simulink model "SystemModel"  (R2026a)
settings: Solver=FixedStepDiscrete  StopTime=inf  FixedStep=ts_system  EnableMultiTasking=on
StartFcn:
  | Simulink.sdi.setRecordData(false);
undefined symbols (not defined in the file): Battery, BCE12, BCE_Set_init, BMS_Controller_State, Cell10_P, Cell11_P, Cell12_P, Cell1_N, Cell1_P, Cell2_P, Cell3_P, Cell4_P, Cell5_P, Cell6_P, Cell7_P, Cell8_P, Cell9_P, Cell_Temperatures, Cell_Voltages, Charging_State, currentFactor, CV_Gain, Device_01, DiscIntNeverNeededParam, I_cc, MaxCellVoltThrsld, noCurrent, Ns_Module, NumModules, OverCellVoltageLimit, sg_bce, SOCInit, SRE, ts_controller, ts_system, UnderCellVoltageLimit, voltThreshold
libraries: slrealtimeethercatlib x99, fl_lib x65, nesl_utility x43, simulink x23, slrealtimeutilitieslib x13, sl_discontinuities x13, dspstat3 x12, canmsglib x11, speedgoatlib_IO611 x9, batt_lib x3, sharedTrackingLibrary x2, BatteryModuleLibrary_12Cells_lib x1
(part 5 of 6)

== system SystemModel/BMS/MIL/Controller/Current Calculations/Discharge_Current_Limit_Calc ==
  MinCellVolt : Inport
  MinCellTemp : Inport  Port=2
  MaxCellTemp : Inport  Port=3
  Divide : Product  Inputs=*/
  Gain : Gain  Gain=-1
  HighTempDchrgCurrentLim : Lookup_n-D  NumberOfTableDimensions=1  BreakpointsForDimension1=273.15+[-30:1:70]  Table=100*(1-tanh(273.15+[-30:1:70]-273.15-50))/2  InternalRulePriority=Speed  RndMeth=Simplest
  InternalCellResistance : Constant  Value=single(max(max(Battery(1).R0_LUT)))  OutDataTypeStr=single  SampleTime=-1
  LowTempDchrgCurrentLim : Lookup_n-D  NumberOfTableDimensions=1  BreakpointsForDimension1=273.15+[-30:1:70]  Table=100*(1+tanh(273.15+[-30:1:70]-(273.15)))/2  InternalRulePriority=Speed  RndMeth=Simplest
  MinMax2 : MinMax  Inputs=3
  Subtract : Sum  Inputs=+-
  UnderVoltageLimit : Constant  Value=UnderCellVoltageLimit  OutDataTypeStr=single  SampleTime=-1
  Discharge_Current_Limit : Outport  VectorParamsAs1DForOutWhenUnconnected=off
  wires:
  MinMax2/1 -> Gain/1  "DischargeCurrentLimit"
  Divide/1 -> MinMax2/1
  MinCellVolt/1 -> Subtract/1
  InternalCellResistance/1 -> Divide/2
  Subtract/1 -> Divide/1
  UnderVoltageLimit/1 -> Subtract/2
  Gain/1 -> Discharge_Current_Limit/1
  MaxCellTemp/1 -> HighTempDchrgCurrentLim/1
  MinCellTemp/1 -> LowTempDchrgCurrentLim/1
  HighTempDchrgCurrentLim/1 -> MinMax2/3
  LowTempDchrgCurrentLim/1 -> MinMax2/2

== system SystemModel/BMS/MIL/Controller/SOC Calculation/Coulomb Counting ==
  Curr : Inport
  Temp : Inport  Port=2
  1-D Lookup Table : Lookup_n-D  NumberOfTableDimensions=1  BreakpointsForDimension1=single(Battery(1).Temperature_LUT)  Table=single(Battery(1).Capacity_LUT)  InternalRulePriority=Speed  RndMeth=Simplest
  Discrete-Time Integrator : DiscreteIntegrator  InitialCondition=single(SOCInit+0.05)  SampleTime=-1  LimitOutput=on  UpperSaturationLimit=1  LowerSaturationLimit=0  ICPrevOutput=DiscIntNeverNeededParam  ICPrevScaledInput=DiscIntNeverNeededParam
  Divide : Product  Inputs=*/
  Gain : Gain  Gain=single(1/3600)
  SOC : Outport  VectorParamsAs1DForOutWhenUnconnected=off
  wires:
  Discrete-Time Integrator/1 -> SOC/1
  Curr/1 -> Gain/1
  Gain/1 -> Divide/1
  Divide/1 -> Discrete-Time Integrator/1
  1-D Lookup Table/1 -> Divide/2  "Capacity"
  Temp/1 -> 1-D Lookup Table/1

== system SystemModel/BMS/MIL/Controller/SOC Calculation/Measurement Function ==
  Current : Inport
  Temperature (K) : Inport  Port=2
  batteryMeasurementFcn : TriggerPort  TriggerType=function-call  IsSimulinkFunction=on  FunctionName=batteryMeasurementFcn  VariantControl=Variant
  Add1 : Sum  Inputs=+--
  Em Table : Lookup_n-D  BreakpointsForDimension1=Battery.SOC_LUT  BreakpointsForDimension2=Battery.Temperature_LUT  BeginIndexSearchUsingPreviousIndexResult=on  Table=Battery.Em_LUT  ExtrapMethod=Clip  InternalRulePriority=Speed  RndMeth=Simplest
      settings: InputPortMap=u0,u1
  Get SOC : Selector  InputPortWidth=2  IndexOptions=Index vector (dialog)  Indices=[1]  OutputSizes=1
  Get U1 : Selector  InputPortWidth=2  IndexOptions=Index vector (dialog)  Indices=2  OutputSizes=1
  Product : Product
  R0 Table : Lookup_n-D  BreakpointsForDimension1=Battery.SOC_LUT  BreakpointsForDimension2=Battery.Temperature_LUT  BeginIndexSearchUsingPreviousIndexResult=on  Table=Battery.R0_LUT  ExtrapMethod=Clip  InternalRulePriority=Speed  RndMeth=Simplest
      settings: InputPortMap=u0,u1
  x : ArgIn  DisableCoverage=on  OutDataTypeStr=single  PortDimensions=2  ArgumentName=x
  y : ArgOut  DisableCoverage=on  OutDataTypeStr=single  ArgumentName=y
  wires:
  Get U1/1 -> Add1/3  "U1"
  Product/1 -> Add1/2
  Current/1 -> Product/2
  R0 Table/1 -> Product/1
  Temperature (K)/1 -> Em Table/2, R0 Table/2
  Add1/1 -> y/1
  Em Table/1 -> Add1/1
  Get SOC/1 -> Em Table/1, R0 Table/1  "SOC"
  x/1 -> Get SOC/1, Get U1/1

== system SystemModel/BMS/MIL/Controller/SOC Calculation/State Transition Function ==
  Current : Inport
  Temperature K : Inport  Port=2
  batteryStateFcn : TriggerPort  TriggerType=function-call  IsSimulinkFunction=on  FunctionName=batteryStateFcn  VariantControl=Variant
  Add : Sum
  Add1 : Sum  Inputs=-+
  C1 : Lookup_n-D  BreakpointsForDimension1=Battery.SOC_LUT  BreakpointsForDimension2=Battery.Temperature_LUT  BeginIndexSearchUsingPreviousIndexResult=on  Table=Battery.C1_LUT  ExtrapMethod=Clip  InternalRulePriority=Speed  RndMeth=Simplest
      settings: InputPortMap=u0,u1
  Constant : Constant  Value=single(ts_system)  OutDataTypeStr=single
  Divide : Product  Inputs=*/
  Divide1 : Product  Inputs=*/
  Divide2 : Product  Inputs=*/
  Gain : Gain  Gain=-3600
  Get SOC : Selector  InputPortWidth=2  IndexOptions=Index vector (dialog)  Indices=1  OutputSizes=1
  Get U1 : Selector  InputPortWidth=2  IndexOptions=Index vector (dialog)  Indices=2  OutputSizes=1
  Lookup Table : Lookup_n-D  NumberOfTableDimensions=1  BreakpointsForDimension1=Battery.Temperature_LUT  BeginIndexSearchUsingPreviousIndexResult=on  Table=Battery.Capacity_LUT  InternalRulePriority=Speed  RndMeth=Simplest
  Mux : Mux  Inputs=2
  Product : Product  OutDataTypeStr=single
  Product1 : Product
  R1 : Lookup_n-D  BreakpointsForDimension1=Battery.SOC_LUT  BreakpointsForDimension2=Battery.Temperature_LUT  BeginIndexSearchUsingPreviousIndexResult=on  Table=Battery.R1_LUT  ExtrapMethod=Clip  InternalRulePriority=Speed  RndMeth=Simplest
      settings: InputPortMap=u0,u1
  x : ArgIn  DisableCoverage=on  OutDataTypeStr=single  PortDimensions=2  ArgumentName=x
  xNext : ArgOut  DisableCoverage=on  OutDataTypeStr=single  PortDimensions=2  ArgumentName=xNext
  wires:
  Lookup Table/1 -> Gain/1  "Cq"
  Product/1 -> Add/2
  Constant/1 -> Product/2
  Current/1 -> Divide1/1, Divide/1  "Current"
  Get SOC/1 -> C1/1, R1/1
  Temperature K/1 -> Lookup Table/1, C1/2, R1/2
  Add/1 -> xNext/1
  x/1 -> Add/1, Get U1/1, Get SOC/1
  Gain/1 -> Divide/2
  Divide/1 -> Mux/1  "xdot_1"
  Get U1/1 -> Divide2/1  "U1"
  Product1/1 -> Divide2/2  "R1*C1"
  R1/1 -> Product1/1  "R1"
  C1/1 -> Product1/2, Divide1/2  "C1"
  Divide1/1 -> Add1/2  "Current/C1"
  Divide2/1 -> Add1/1
  Add1/1 -> Mux/2  "xdot_2"
  Mux/1 -> Product/1  "xdot"

== system SystemModel/BMS/MIL/Controller/SOC Calculation/UKF_EKF_1TC ==
  Cell_Voltage : Inport
  Enable : EnablePort
  EKF : sharedTrackingLibrary/Extended Kalman Filter  StateTransitionFcn=batteryStateFcn  HasStateTransitionJacobianFcn=off  HasAdditiveProcessNoise=Additive  ProcessNoise=1e-10*eye(2)  HasTimeVaryingProcessNoise=off  HasStateTransitionFcnExtraArgument=0  InitialState=[single(SOCInit+0.05); 0;]  InitialStateCovariance=[1e-5 1]  MeasurementFcn1=batteryMeasurementFcn  HasMeasurementJacobianFcn1=off  HasMeasurementEnablePort1=off  HasAdditiveMeasurementNoise1=Additive  MeasurementNoise1=1e-1  HasTimeVaryingMeasurementNoise1=off  HasMeasurementFcnExtraArgument1=0  HasMeasurementWrapping1=off  MeasurementFcn2=myMeasurementFcn  HasMeasurementJacobianFcn2=off  HasMeasurementEnablePort2=off  HasAdditiveMeasurementNoise2=Additive  MeasurementNoise2=1  HasTimeVaryingMeasurementNoise2=off  HasMeasurementFcnExtraArgument2=0  HasMeasurementWrapping2=off  MeasurementFcn3=myMeasurementFcn  HasMeasurementJacobianFcn3=off  HasMeasurementEnablePort3=off  HasAdditiveMeasurementNoise3=Additive  MeasurementNoise3=1  HasTimeVaryingMeasurementNoise3=off  HasMeasurementFcnExtraArgument3=0  HasMeasurementWrapping3=off  MeasurementFcn4=myMeasurementFcn  HasMeasurementJacobianFcn4=off  HasMeasurementEnablePort4=off  HasAdditiveMeasurementNoise4=Additive  MeasurementNoise4=1  HasTimeVaryingMeasurementNoise4=off  HasMeasurementFcnExtraArgument4=0  HasMeasurementWrapping4=off  MeasurementFcn5=myMeasurementFcn  HasMeasurementJacobianFcn5=off  HasMeasurementEnablePort5=off  HasAdditiveMeasurementNoise5=Additive  MeasurementNoise5=1  HasTimeVaryingMeasurementNoise5=off  HasMeasurementFcnExtraArgument5=0  HasMeasurementWrapping5=off  EnableMultirate=off  StateTransitionFcnSampleTime=1  MeasurementFcn1SampleTime=1  MeasurementFcn2SampleTime=1  MeasurementFcn3SampleTime=1  MeasurementFcn4SampleTime=1  MeasurementFcn5SampleTime=1  UseCurrentEstimator=on  OutputStateCovariance=off  DataType=single  SampleTime=ts_controller  NumberOfMeasurements=1
  SOC : Selector  InputPortWidth=2  IndexOptions=Index vector (dialog)  Indices=1  OutputSizes=1
  SOC1 : Selector  InputPortWidth=2  IndexOptions=Index vector (dialog)  Indices=1  OutputSizes=1
  UKF : sharedTrackingLibrary/Unscented Kalman Filter  StateTransitionFcn=batteryStateFcn  HasAdditiveProcessNoise=Additive  ProcessNoise=1e-10*eye(2)  HasTimeVaryingProcessNoise=off  HasStateTransitionFcnExtraArgument=0  InitialState=[single(SOCInit+0.05); 0;]  InitialStateCovariance=[1e-5 1]  Alpha=1  Beta=2  Kappa=1  MeasurementFcn1=batteryMeasurementFcn  HasMeasurementEnablePort1=off  HasAdditiveMeasurementNoise1=Additive  MeasurementNoise1=0.1  HasTimeVaryingMeasurementNoise1=off  HasMeasurementFcnExtraArgument1=0  HasMeasurementWrapping1=off  MeasurementFcn2=myMeasurementFcn  HasMeasurementEnablePort2=off  HasAdditiveMeasurementNoise2=Additive  MeasurementNoise2=1  HasTimeVaryingMeasurementNoise2=off  HasMeasurementFcnExtraArgument2=0  HasMeasurementWrapping2=off  MeasurementFcn3=myMeasurementFcn  HasMeasurementEnablePort3=off  HasAdditiveMeasurementNoise3=Additive  MeasurementNoise3=1  HasTimeVaryingMeasurementNoise3=off  HasMeasurementFcnExtraArgument3=0  HasMeasurementWrapping3=off  MeasurementFcn4=myMeasurementFcn  HasMeasurementEnablePort4=off  HasAdditiveMeasurementNoise4=Additive  MeasurementNoise4=1  HasTimeVaryingMeasurementNoise4=off  HasMeasurementFcnExtraArgument4=0  HasMeasurementWrapping4=off  MeasurementFcn5=myMeasurementFcn  HasMeasurementEnablePort5=off  HasAdditiveMeasurementNoise5=Additive  MeasurementNoise5=1  HasTimeVaryingMeasurementNoise5=off  HasMeasurementFcnExtraArgument5=0  HasMeasurementWrapping5=off  EnableMultirate=off  StateTransitionFcnSampleTime=-1  MeasurementFcn1SampleTime=-1  MeasurementFcn2SampleTime=-1  MeasurementFcn3SampleTime=-1  MeasurementFcn4SampleTime=-1  MeasurementFcn5SampleTime=-1  UseCurrentEstimator=on  OutputStateCovariance=off  DataType=single  SampleTime=ts_controller  NumberOfMeasurements=1
  SOC_UKF : Outport  VectorParamsAs1DForOutWhenUnconnected=off
  SOC_EKF : Outport  Port=2  VectorParamsAs1DForOutWhenUnconnected=off
  wires:
  UKF/1 -> SOC1/1
  Cell_Voltage/1 -> UKF/1, EKF/1
  SOC1/1 -> SOC_UKF/1  "SOC_UKF"
  EKF/1 -> SOC/1
  SOC/1 -> SOC_EKF/1  "SOC_EKF"

== system SystemModel/Battery/Bypass/Bypass Values/12-Cell/Celsius_to_Kelvin ==
  C : Inport
  Add : Sum
  Constant : Constant  Value=273.15  SampleTime=-1
  Data Type Conversion3 : DataTypeConversion  OutDataTypeStr=single  SaturateOnIntegerOverflow=off  RndMeth=Floor
  K : Outport
  wires:
  Constant/1 -> Add/2
  Add/1 -> Data Type Conversion3/1
  C/1 -> Add/1
  Data Type Conversion3/1 -> K/1  "LowTempLimit"

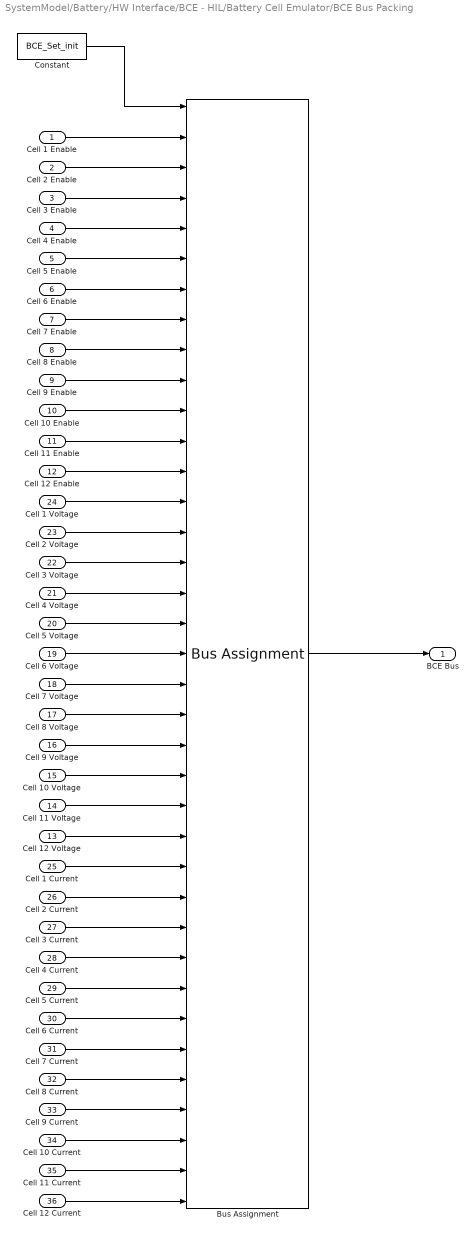
== system SystemModel/Battery/HW Interface/BCE - HIL/Battery Cell Emulator/BCE Bus Packing  ==
  Cell 1 Enable : Inport
  Cell 2 Enable : Inport  Port=2
  Cell 3 Enable : Inport  Port=3
  Cell 4 Enable : Inport  Port=4
  Cell 5 Enable : Inport  Port=5
  Cell 6 Enable : Inport  Port=6
  Cell 7 Enable : Inport  Port=7
  Cell 8 Enable : Inport  Port=8
  Cell 9 Enable : Inport  Port=9
  Cell 10 Enable : Inport  Port=10
  Cell 11 Enable : Inport  Port=11
  Cell 12 Enable : Inport  Port=12
  Cell 12 Voltage : Inport  Port=13
  Cell 11 Voltage : Inport  Port=14
  Cell 10 Voltage : Inport  Port=15
  Cell 9 Voltage : Inport  Port=16
  Cell 8 Voltage : Inport  Port=17
  Cell 7 Voltage : Inport  Port=18
  Cell 6 Voltage : Inport  Port=19
  Cell 5 Voltage : Inport  Port=20
  Cell 4 Voltage : Inport  Port=21
  Cell 3 Voltage : Inport  Port=22
  Cell 2 Voltage : Inport  Port=23
  Cell 1 Voltage : Inport  Port=24
  Cell 1 Current : Inport  Port=25
  Cell 2 Current : Inport  Port=26
  Cell 3 Current : Inport  Port=27
  Cell 4 Current : Inport  Port=28
  Cell 5 Current : Inport  Port=29
  Cell 6 Current : Inport  Port=30
  Cell 7 Current : Inport  Port=31
  Cell 8 Current : Inport  Port=32
  Cell 9 Current : Inport  Port=33
  Cell 10 Current : Inport  Port=34
  Cell 11 Current : Inport  Port=35
  Cell 12 Current : Inport  Port=36
  Bus Assignment : BusAssignment  AssignedSignals=Cell_1.Enable,Cell_2.Enable,Cell_3.Enable,Cell_4.Enable,Cell_5.Enable,Cell_6.Enable,Cell_7.Enable,Cell_8.Enable,Cell_9.Enable,Cell_10.Enable,Cell_11.Enable,Cell_12.Enable,Cell_1.V,Cell_2.V,Cell_3.V,Cell_4.V,Cell_5.V,Cell_6.V,Cell_7.V,Cell_8.V,Cell_9.V,Cell_10.V,Cell_11.V,Cell_12.V,Cell_1.I,Cell_2.I,Cell_3.I,Cell_4.I,Cell_5.I,Cell_6.I,Cell_7.I,Cell_8.I,Cell_9.I,Cell_10.I,Cell_11.I,Cell_12.I
  Constant : Constant  Value=BCE_Set_init  OutDataTypeStr=Bus: BCE_Set
  BCE Bus : Outport
  wires:
  Cell 11 Enable/1 -> Bus Assignment/12
  Cell 11 Voltage/1 -> Bus Assignment/24
  Cell 11 Current/1 -> Bus Assignment/36
  Cell 12 Current/1 -> Bus Assignment/37
  Cell 12 Voltage/1 -> Bus Assignment/25
  Cell 12 Enable/1 -> Bus Assignment/13
  Cell 10 Enable/1 -> Bus Assignment/11
  Cell 10 Voltage/1 -> Bus Assignment/23
  Cell 10 Current/1 -> Bus Assignment/35
  Cell 9 Current/1 -> Bus Assignment/34
  Cell 9 Voltage/1 -> Bus Assignment/22
  Cell 9 Enable/1 -> Bus Assignment/10
  Cell 5 Enable/1 -> Bus Assignment/6
  Cell 5 Voltage/1 -> Bus Assignment/18
  Cell 5 Current/1 -> Bus Assignment/30
  Cell 6 Current/1 -> Bus Assignment/31
  Cell 6 Voltage/1 -> Bus Assignment/19
  Cell 6 Enable/1 -> Bus Assignment/7
  Cell 8 Enable/1 -> Bus Assignment/9
  Cell 8 Voltage/1 -> Bus Assignment/21
  Cell 8 Current/1 -> Bus Assignment/33
  Cell 7 Current/1 -> Bus Assignment/32
  Cell 7 Voltage/1 -> Bus Assignment/20
  Cell 7 Enable/1 -> Bus Assignment/8
  Cell 3 Enable/1 -> Bus Assignment/4
  Cell 3 Voltage/1 -> Bus Assignment/16
  Cell 3 Current/1 -> Bus Assignment/28
  Cell 4 Current/1 -> Bus Assignment/29
  Cell 4 Voltage/1 -> Bus Assignment/17
  Cell 4 Enable/1 -> Bus Assignment/5
  Cell 2 Enable/1 -> Bus Assignment/3
  Cell 2 Voltage/1 -> Bus Assignment/15
  Cell 2 Current/1 -> Bus Assignment/27
  Cell 1 Current/1 -> Bus Assignment/26
  Cell 1 Enable/1 -> Bus Assignment/2
  Bus Assignment/1 -> BCE Bus/1
  Constant/1 -> Bus Assignment/1
  Cell 1 Voltage/1 -> Bus Assignment/14

== system SystemModel/Battery/HW Interface/BCE - HIL/Battery Cell Emulator/BCE Read  ==
  Subsystem : Subsystem
  Data : Outport  OutDataTypeStr=Bus: BCE_Get
  wires:
  Subsystem/1(Data) -> Data/1

== system SystemModel/Battery/HW Interface/BCE - HIL/Battery Cell Emulator/BCE Setup  ==
  EtherCAT Init : slrealtimeethercatlib/EtherCAT Init  Priority=0  config_file=C:\Users\jatin.anand\AppData\Local\Temp\sg_bmts\SystemModel\sg_bmts_ENI_bus0.xml  device_id=0  portnum=1  initstate=2  dctuning=0  enaDebug=0  logFile='c:\dbglog.txt'  sample_time=0.001000  DCMode=0
  Terminator : Terminator
  wires:
  EtherCAT Init/1 -> Terminator/1

== system SystemModel/Battery/HW Interface/BCE - HIL/Battery Cell Emulator/BCE Write  ==
  Data : Inport  OutDataTypeStr=Bus: BCE_Set
  Subsystem : Subsystem
  wires:
  Data/1 -> Subsystem/1(Data)

== system SystemModel/Battery/HW Interface/BCE - HIL/Battery Cell Emulator/BCE Read /Subsystem ==
  "BCE Read " : Subsystem
  Data : Outport  OutDataTypeStr=Bus: BCE_Get
  wires:
  "BCE Read "/1(Data) -> Data/1

== system SystemModel/Battery/HW Interface/BCE - HIL/Battery Cell Emulator/BCE Write /Subsystem ==
  Data : Inport  OutDataTypeStr=Bus: BCE_Set
  "BCE Write " : Subsystem
  wires:
  Data/1 -> "BCE Write "/1(Data)

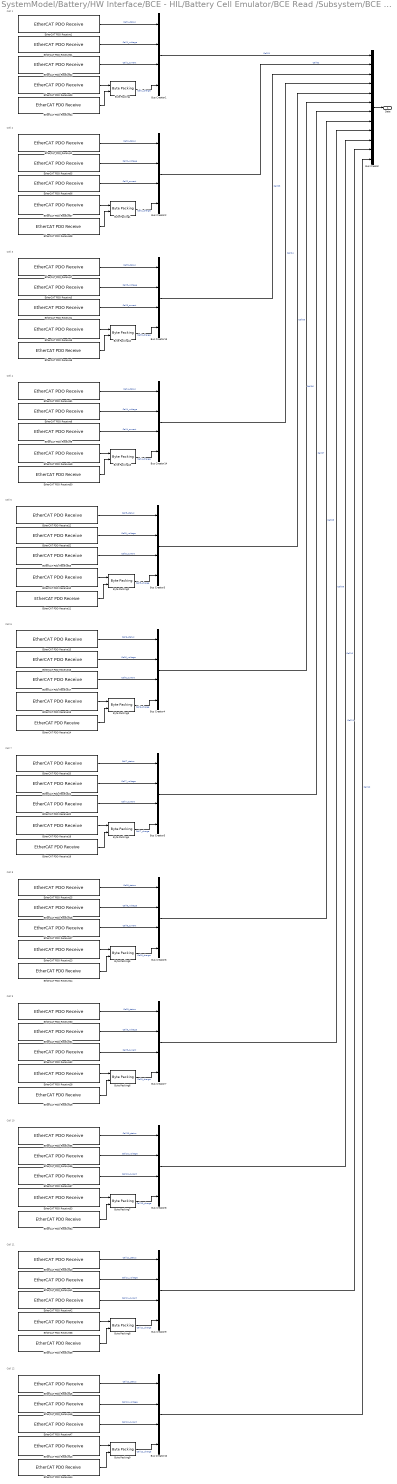
== system SystemModel/Battery/HW Interface/BCE - HIL/Battery Cell Emulator/BCE Read /Subsystem/BCE Read  ==
  note: Cell 7
  note: Cell 2
  note: Cell 6
  note: Cell 8
  note: Cell 12
  note: Cell 11
  note: Cell 3
  note: Cell 5
  note: Cell 4
  note: Cell 10
  note: Cell 9
  note: Cell 1
  Bus Creator : BusCreator  Inputs=12  OutDataTypeStr=Bus: BCE_Get
      settings: InheritFromInputs=off
  Bus Creator{1..10,13..14} (12 alike) : BusCreator  Inputs=4  OutDataTypeStr=Bus: Cell_Get
      settings: InheritFromInputs=off
  Byte Packing{,1..9,12..13} (12 alike) : slrealtimeutilitieslib/Byte Packing  MaskPackedDataType=uint64  MaskUnpackedDataTypes={'uint32','uint32'}  MaskAlignment=1
  EtherCAT PDO Receive01 : slrealtimeethercatlib/EtherCAT PDO Receive  Priority=2  sig_name=Device_01 (BCE12-0505).Tx_Cell_01.voltage  sig_offset=16  sig_type=single  type_size=32  sig_dim=1  device_id=0  sample_time=0.001000
  EtherCAT PDO Receive02 : slrealtimeethercatlib/EtherCAT PDO Receive  Priority=2  sig_name=Device_01 (BCE12-0505).Tx_Cell_01.current  sig_offset=48  sig_type=single  type_size=32  sig_dim=1  device_id=0  sample_time=0.001000
  EtherCAT PDO Receive03 : slrealtimeethercatlib/EtherCAT PDO Receive  Priority=2  sig_name=Device_01 (BCE12-0505).Tx_Cell_01.chargeMSB  sig_offset=80  sig_type=uint32  type_size=32  sig_dim=1  device_id=0  sample_time=0.001000
  EtherCAT PDO Receive04 : slrealtimeethercatlib/EtherCAT PDO Receive  Priority=2  sig_name=Device_01 (BCE12-0505).Tx_Cell_01.chargeLSB  sig_offset=112  sig_type=uint32  type_size=32  sig_dim=1  device_id=0  sample_time=0.001000
  EtherCAT PDO Receive05 : slrealtimeethercatlib/EtherCAT PDO Receive  Priority=2  sig_name=Device_01 (BCE12-0505).Tx_Cell_02.voltage  sig_offset=160  sig_type=single  type_size=32  sig_dim=1  device_id=0  sample_time=0.001000
  EtherCAT PDO Receive06 : slrealtimeethercatlib/EtherCAT PDO Receive  Priority=2  sig_name=Device_01 (BCE12-0505).Tx_Cell_02.current  sig_offset=192  sig_type=single  type_size=32  sig_dim=1  device_id=0  sample_time=0.001000
  EtherCAT PDO Receive07 : slrealtimeethercatlib/EtherCAT PDO Receive  Priority=2  sig_name=Device_01 (BCE12-0505).Tx_Cell_02.chargeMSB  sig_offset=224  sig_type=uint32  type_size=32  sig_dim=1  device_id=0  sample_time=0.001000
  EtherCAT PDO Receive08 : slrealtimeethercatlib/EtherCAT PDO Receive  Priority=2  sig_name=Device_01 (BCE12-0505).Tx_Cell_02.chargeLSB  sig_offset=256  sig_type=uint32  type_size=32  sig_dim=1  device_id=0  sample_time=0.001000
  EtherCAT PDO Receive1 : slrealtimeethercatlib/EtherCAT PDO Receive  Priority=2  sig_name=Device_01 (BCE12-0505).Tx_Cell_01.status  sig_offset=0  sig_type=uint16  type_size=16  sig_dim=1  device_id=0  sample_time=0.001000
  EtherCAT PDO Receive10 : slrealtimeethercatlib/EtherCAT PDO Receive  Priority=2  sig_name=Device_01 (BCE12-0505).Tx_Cell_05.chargeMSB  sig_offset=656  sig_type=uint32  type_size=32  sig_dim=1  device_id=0  sample_time=0.001000
  EtherCAT PDO Receive11 : slrealtimeethercatlib/EtherCAT PDO Receive  Priority=2  sig_name=Device_01 (BCE12-0505).Tx_Cell_05.chargeLSB  sig_offset=688  sig_type=uint32  type_size=32  sig_dim=1  device_id=0  sample_time=0.001000
  EtherCAT PDO Receive12 : slrealtimeethercatlib/EtherCAT PDO Receive  Priority=2  sig_name=Device_01 (BCE12-0505).Tx_Cell_05.status  sig_offset=576  sig_type=uint16  type_size=16  sig_dim=1  device_id=0  sample_time=0.001000
  EtherCAT PDO Receive13 : slrealtimeethercatlib/EtherCAT PDO Receive  Priority=2  sig_name=Device_01 (BCE12-0505).Tx_Cell_06.chargeMSB  sig_offset=800  sig_type=uint32  type_size=32  sig_dim=1  device_id=0  sample_time=0.001000
  EtherCAT PDO Receive14 : slrealtimeethercatlib/EtherCAT PDO Receive  Priority=2  sig_name=Device_01 (BCE12-0505).Tx_Cell_06.chargeLSB  sig_offset=832  sig_type=uint32  type_size=32  sig_dim=1  device_id=0  sample_time=0.001000
  EtherCAT PDO Receive15 : slrealtimeethercatlib/EtherCAT PDO Receive  Priority=2  sig_name=Device_01 (BCE12-0505).Tx_Cell_06.status  sig_offset=720  sig_type=uint16  type_size=16  sig_dim=1  device_id=0  sample_time=0.001000
  EtherCAT PDO Receive16 : slrealtimeethercatlib/EtherCAT PDO Receive  Priority=2  sig_name=Device_01 (BCE12-0505).Tx_Cell_06.voltage  sig_offset=736  sig_type=single  type_size=32  sig_dim=1  device_id=0  sample_time=0.001000
  EtherCAT PDO Receive17 : slrealtimeethercatlib/EtherCAT PDO Receive  Priority=2  sig_name=Device_01 (BCE12-0505).Tx_Cell_06.current  sig_offset=768  sig_type=single  type_size=32  sig_dim=1  device_id=0  sample_time=0.001000
  EtherCAT PDO Receive18 : slrealtimeethercatlib/EtherCAT PDO Receive  Priority=2  sig_name=Device_01 (BCE12-0505).Tx_Cell_07.chargeMSB  sig_offset=944  sig_type=uint32  type_size=32  sig_dim=1  device_id=0  sample_time=0.001000
  EtherCAT PDO Receive19 : slrealtimeethercatlib/EtherCAT PDO Receive  Priority=2  sig_name=Device_01 (BCE12-0505).Tx_Cell_07.chargeLSB  sig_offset=976  sig_type=uint32  type_size=32  sig_dim=1  device_id=0  sample_time=0.001000
  EtherCAT PDO Receive2 : slrealtimeethercatlib/EtherCAT PDO Receive  Priority=2  sig_name=Device_01 (BCE12-0505).Tx_Cell_02.status  sig_offset=144  sig_type=uint16  type_size=16  sig_dim=1  device_id=0  sample_time=0.001000
  EtherCAT PDO Receive20 : slrealtimeethercatlib/EtherCAT PDO Receive  Priority=2  sig_name=Device_01 (BCE12-0505).Tx_Cell_07.status  sig_offset=864  sig_type=uint16  type_size=16  sig_dim=1  device_id=0  sample_time=0.001000
  EtherCAT PDO Receive21 : slrealtimeethercatlib/EtherCAT PDO Receive  Priority=2  sig_name=Device_01 (BCE12-0505).Tx_Cell_07.voltage  sig_offset=880  sig_type=single  type_size=32  sig_dim=1  device_id=0  sample_time=0.001000
  EtherCAT PDO Receive22 : slrealtimeethercatlib/EtherCAT PDO Receive  Priority=2  sig_name=Device_01 (BCE12-0505).Tx_Cell_07.current  sig_offset=912  sig_type=single  type_size=32  sig_dim=1  device_id=0  sample_time=0.001000
  EtherCAT PDO Receive23 : slrealtimeethercatlib/EtherCAT PDO Receive  Priority=2  sig_name=Device_01 (BCE12-0505).Tx_Cell_08.chargeMSB  sig_offset=1088  sig_type=uint32  type_size=32  sig_dim=1  device_id=0  sample_time=0.001000
  EtherCAT PDO Receive24 : slrealtimeethercatlib/EtherCAT PDO Receive  Priority=2  sig_name=Device_01 (BCE12-0505).Tx_Cell_08.chargeLSB  sig_offset=1120  sig_type=uint32  type_size=32  sig_dim=1  device_id=0  sample_time=0.001000
  EtherCAT PDO Receive25 : slrealtimeethercatlib/EtherCAT PDO Receive  Priority=2  sig_name=Device_01 (BCE12-0505).Tx_Cell_08.status  sig_offset=1008  sig_type=uint16  type_size=16  sig_dim=1  device_id=0  sample_time=0.001000
  EtherCAT PDO Receive26 : slrealtimeethercatlib/EtherCAT PDO Receive  Priority=2  sig_name=Device_01 (BCE12-0505).Tx_Cell_08.voltage  sig_offset=1024  sig_type=single  type_size=32  sig_dim=1  device_id=0  sample_time=0.001000
  EtherCAT PDO Receive27 : slrealtimeethercatlib/EtherCAT PDO Receive  Priority=2  sig_name=Device_01 (BCE12-0505).Tx_Cell_08.current  sig_offset=1056  sig_type=single  type_size=32  sig_dim=1  device_id=0  sample_time=0.001000
  EtherCAT PDO Receive28 : slrealtimeethercatlib/EtherCAT PDO Receive  Priority=2  sig_name=Device_01 (BCE12-0505).Tx_Cell_09.chargeMSB  sig_offset=1232  sig_type=uint32  type_size=32  sig_dim=1  device_id=0  sample_time=0.001000
  EtherCAT PDO Receive29 : slrealtimeethercatlib/EtherCAT PDO Receive  Priority=2  sig_name=Device_01 (BCE12-0505).Tx_Cell_09.chargeLSB  sig_offset=1264  sig_type=uint32  type_size=32  sig_dim=1  device_id=0  sample_time=0.001000
  EtherCAT PDO Receive3 : slrealtimeethercatlib/EtherCAT PDO Receive  Priority=2  sig_name=Device_01 (BCE12-0505).Tx_Cell_03.voltage  sig_offset=304  sig_type=single  type_size=32  sig_dim=1  device_id=0  sample_time=0.001000
  EtherCAT PDO Receive30 : slrealtimeethercatlib/EtherCAT PDO Receive  Priority=2  sig_name=Device_01 (BCE12-0505).Tx_Cell_09.status  sig_offset=1152  sig_type=uint16  type_size=16  sig_dim=1  device_id=0  sample_time=0.001000
  EtherCAT PDO Receive31 : slrealtimeethercatlib/EtherCAT PDO Receive  Priority=2  sig_name=Device_01 (BCE12-0505).Tx_Cell_09.voltage  sig_offset=1168  sig_type=single  type_size=32  sig_dim=1  device_id=0  sample_time=0.001000
  EtherCAT PDO Receive32 : slrealtimeethercatlib/EtherCAT PDO Receive  Priority=2  sig_name=Device_01 (BCE12-0505).Tx_Cell_09.current  sig_offset=1200  sig_type=single  type_size=32  sig_dim=1  device_id=0  sample_time=0.001000
  EtherCAT PDO Receive33 : slrealtimeethercatlib/EtherCAT PDO Receive  Priority=2  sig_name=Device_01 (BCE12-0505).Tx_Cell_10.chargeMSB  sig_offset=1376  sig_type=uint32  type_size=32  sig_dim=1  device_id=0  sample_time=0.001000
  EtherCAT PDO Receive34 : slrealtimeethercatlib/EtherCAT PDO Receive  Priority=2  sig_name=Device_01 (BCE12-0505).Tx_Cell_10.chargeLSB  sig_offset=1408  sig_type=uint32  type_size=32  sig_dim=1  device_id=0  sample_time=0.001000
  EtherCAT PDO Receive35 : slrealtimeethercatlib/EtherCAT PDO Receive  Priority=2  sig_name=Device_01 (BCE12-0505).Tx_Cell_10.status  sig_offset=1296  sig_type=uint16  type_size=16  sig_dim=1  device_id=0  sample_time=0.001000
  EtherCAT PDO Receive36 : slrealtimeethercatlib/EtherCAT PDO Receive  Priority=2  sig_name=Device_01 (BCE12-0505).Tx_Cell_10.voltage  sig_offset=1312  sig_type=single  type_size=32  sig_dim=1  device_id=0  sample_time=0.001000
  EtherCAT PDO Receive37 : slrealtimeethercatlib/EtherCAT PDO Receive  Priority=2  sig_name=Device_01 (BCE12-0505).Tx_Cell_10.current  sig_offset=1344  sig_type=single  type_size=32  sig_dim=1  device_id=0  sample_time=0.001000
  EtherCAT PDO Receive38 : slrealtimeethercatlib/EtherCAT PDO Receive  Priority=2  sig_name=Device_01 (BCE12-0505).Tx_Cell_11.chargeMSB  sig_offset=1520  sig_type=uint32  type_size=32  sig_dim=1  device_id=0  sample_time=0.001000
  EtherCAT PDO Receive39 : slrealtimeethercatlib/EtherCAT PDO Receive  Priority=2  sig_name=Device_01 (BCE12-0505).Tx_Cell_11.chargeLSB  sig_offset=1552  sig_type=uint32  type_size=32  sig_dim=1  device_id=0  sample_time=0.001000
  EtherCAT PDO Receive4 : slrealtimeethercatlib/EtherCAT PDO Receive  Priority=2  sig_name=Device_01 (BCE12-0505).Tx_Cell_03.current  sig_offset=336  sig_type=single  type_size=32  sig_dim=1  device_id=0  sample_time=0.001000
  EtherCAT PDO Receive40 : slrealtimeethercatlib/EtherCAT PDO Receive  Priority=2  sig_name=Device_01 (BCE12-0505).Tx_Cell_11.status  sig_offset=1440  sig_type=uint16  type_size=16  sig_dim=1  device_id=0  sample_time=0.001000
  EtherCAT PDO Receive41 : slrealtimeethercatlib/EtherCAT PDO Receive  Priority=2  sig_name=Device_01 (BCE12-0505).Tx_Cell_11.voltage  sig_offset=1456  sig_type=single  type_size=32  sig_dim=1  device_id=0  sample_time=0.001000
  EtherCAT PDO Receive42 : slrealtimeethercatlib/EtherCAT PDO Receive  Priority=2  sig_name=Device_01 (BCE12-0505).Tx_Cell_11.current  sig_offset=1488  sig_type=single  type_size=32  sig_dim=1  device_id=0  sample_time=0.001000
  EtherCAT PDO Receive43 : slrealtimeethercatlib/EtherCAT PDO Receive  Priority=2  sig_name=Device_01 (BCE12-0505).Tx_Cell_12.chargeMSB  sig_offset=1664  sig_type=uint32  type_size=32  sig_dim=1  device_id=0  sample_time=0.001000
  EtherCAT PDO Receive44 : slrealtimeethercatlib/EtherCAT PDO Receive  Priority=2  sig_name=Device_01 (BCE12-0505).Tx_Cell_12.chargeLSB  sig_offset=1696  sig_type=uint32  type_size=32  sig_dim=1  device_id=0  sample_time=0.001000
  EtherCAT PDO Receive45 : slrealtimeethercatlib/EtherCAT PDO Receive  Priority=2  sig_name=Device_01 (BCE12-0505).Tx_Cell_12.status  sig_offset=1584  sig_type=uint16  type_size=16  sig_dim=1  device_id=0  sample_time=0.001000
  EtherCAT PDO Receive46 : slrealtimeethercatlib/EtherCAT PDO Receive  Priority=2  sig_name=Device_01 (BCE12-0505).Tx_Cell_12.voltage  sig_offset=1600  sig_type=single  type_size=32  sig_dim=1  device_id=0  sample_time=0.001000
  EtherCAT PDO Receive47 : slrealtimeethercatlib/EtherCAT PDO Receive  Priority=2  sig_name=Device_01 (BCE12-0505).Tx_Cell_12.current  sig_offset=1632  sig_type=single  type_size=32  sig_dim=1  device_id=0  sample_time=0.001000
  EtherCAT PDO Receive49 : slrealtimeethercatlib/EtherCAT PDO Receive  Priority=2  sig_name=Device_01 (BCE12-0505).Tx_Cell_04.chargeMSB  sig_offset=512  sig_type=uint32  type_size=32  sig_dim=1  device_id=0  sample_time=0.001000
  EtherCAT PDO Receive5 : slrealtimeethercatlib/EtherCAT PDO Receive  Priority=2  sig_name=Device_01 (BCE12-0505).Tx_Cell_03.chargeMSB  sig_offset=368  sig_type=uint32  type_size=32  sig_dim=1  device_id=0  sample_time=0.001000
  EtherCAT PDO Receive50 : slrealtimeethercatlib/EtherCAT PDO Receive  Priority=2  sig_name=Device_01 (BCE12-0505).Tx_Cell_04.chargeLSB  sig_offset=544  sig_type=uint32  type_size=32  sig_dim=1  device_id=0  sample_time=0.001000
  EtherCAT PDO Receive51 : slrealtimeethercatlib/EtherCAT PDO Receive  Priority=2  sig_name=Device_01 (BCE12-0505).Tx_Cell_04.status  sig_offset=432  sig_type=uint16  type_size=16  sig_dim=1  device_id=0  sample_time=0.001000
  EtherCAT PDO Receive52 : slrealtimeethercatlib/EtherCAT PDO Receive  Priority=2  sig_name=Device_01 (BCE12-0505).Tx_Cell_05.voltage  sig_offset=592  sig_type=single  type_size=32  sig_dim=1  device_id=0  sample_time=0.001000
  EtherCAT PDO Receive53 : slrealtimeethercatlib/EtherCAT PDO Receive  Priority=2  sig_name=Device_01 (BCE12-0505).Tx_Cell_05.current  sig_offset=624  sig_type=single  type_size=32  sig_dim=1  device_id=0  sample_time=0.001000
  EtherCAT PDO Receive6 : slrealtimeethercatlib/EtherCAT PDO Receive  Priority=2  sig_name=Device_01 (BCE12-0505).Tx_Cell_03.chargeLSB  sig_offset=400  sig_type=uint32  type_size=32  sig_dim=1  device_id=0  sample_time=0.001000
  EtherCAT PDO Receive7 : slrealtimeethercatlib/EtherCAT PDO Receive  Priority=2  sig_name=Device_01 (BCE12-0505).Tx_Cell_03.status  sig_offset=288  sig_type=uint16  type_size=16  sig_dim=1  device_id=0  sample_time=0.001000
  EtherCAT PDO Receive8 : slrealtimeethercatlib/EtherCAT PDO Receive  Priority=2  sig_name=Device_01 (BCE12-0505).Tx_Cell_04.voltage  sig_offset=448  sig_type=single  type_size=32  sig_dim=1  device_id=0  sample_time=0.001000
  EtherCAT PDO Receive9 : slrealtimeethercatlib/EtherCAT PDO Receive  Priority=2  sig_name=Device_01 (BCE12-0505).Tx_Cell_04.current  sig_offset=480  sig_type=single  type_size=32  sig_dim=1  device_id=0  sample_time=0.001000
  Data : Outport  OutDataTypeStr=Bus: BCE_Get
  wires:
  EtherCAT PDO Receive04/1 -> Byte Packing/2
  EtherCAT PDO Receive53/1 -> Bus Creator3/3  "Cell5_current"
  Bus Creator7/1 -> Bus Creator/9  "Cell09"
  EtherCAT PDO Receive1/1 -> Bus Creator1/1  "Cell1_status"
  EtherCAT PDO Receive40/1 -> Bus Creator9/1  "Cell11_status"
  EtherCAT PDO Receive39/1 -> Byte Packing8/2
  EtherCAT PDO Receive18/1 -> Byte Packing4/1
  Byte Packing13/1 -> Bus Creator14/4  "Cell4_charge"
  Bus Creator14/1 -> Bus Creator/4  "Cell04"
  EtherCAT PDO Receive21/1 -> Bus Creator5/2  "Cell7_voltage"
  EtherCAT PDO Receive52/1 -> Bus Creator3/2  "Cell5_voltage"
  EtherCAT PDO Receive15/1 -> Bus Creator4/1  "Cell6_status"
  EtherCAT PDO Receive11/1 -> Byte Packing2/2
  EtherCAT PDO Receive26/1 -> Bus Creator6/2  "Cell8_voltage"
  EtherCAT PDO Receive33/1 -> Byte Packing7/1
  EtherCAT PDO Receive12/1 -> Bus Creator3/1  "Cell5_status"
  Byte Packing2/1 -> Bus Creator3/4  "Cell5_charge"
  Byte Packing4/1 -> Bus Creator5/4  "Cell7_charge"
  Byte Packing6/1 -> Bus Creator7/4  "Cell9_charge"
  EtherCAT PDO Receive7/1 -> Bus Creator13/1  "Cell3_status"
  Bus Creator4/1 -> Bus Creator/6  "Cell06"
  Bus Creator6/1 -> Bus Creator/8  "Cell08"
  EtherCAT PDO Receive30/1 -> Bus Creator7/1  "Cell9_status"
  EtherCAT PDO Receive4/1 -> Bus Creator13/3  "Cell3_current"
  Bus Creator13/1 -> Bus Creator/3  "Cell03"
  Byte Packing7/1 -> Bus Creator8/4  "Cell10_charge"
  EtherCAT PDO Receive01/1 -> Bus Creator1/2  "Cell1_voltage"
  EtherCAT PDO Receive35/1 -> Bus Creator8/1  "Cell10_status"
  EtherCAT PDO Receive29/1 -> Byte Packing6/2
  EtherCAT PDO Receive27/1 -> Bus Creator6/3  "Cell8_current"
  EtherCAT PDO Receive32/1 -> Bus Creator7/3  "Cell9_current"
  EtherCAT PDO Receive41/1 -> Bus Creator9/2  "Cell11_voltage"
  EtherCAT PDO Receive5/1 -> Byte Packing12/1
  EtherCAT PDO Receive3/1 -> Bus Creator13/2  "Cell3_voltage"
  EtherCAT PDO Receive46/1 -> Bus Creator10/2  "Cell12_voltage"
  EtherCAT PDO Receive6/1 -> Byte Packing12/2
  EtherCAT PDO Receive17/1 -> Bus Creator4/3  "Cell6_current"
  EtherCAT PDO Receive9/1 -> Bus Creator14/3  "Cell4_current"
  Bus Creator9/1 -> Bus Creator/11  "Cell11"
  EtherCAT PDO Receive43/1 -> Byte Packing9/1
  EtherCAT PDO Receive44/1 -> Byte Packing9/2
  EtherCAT PDO Receive45/1 -> Bus Creator10/1  "Cell12_status"
  EtherCAT PDO Receive23/1 -> Byte Packing5/1
  EtherCAT PDO Receive37/1 -> Bus Creator8/3  "Cell10_current"
  EtherCAT PDO Receive8/1 -> Bus Creator14/2  "Cell4_voltage"
  EtherCAT PDO Receive14/1 -> Byte Packing3/2
  EtherCAT PDO Receive49/1 -> Byte Packing13/1
  EtherCAT PDO Receive19/1 -> Byte Packing4/2
  EtherCAT PDO Receive24/1 -> Byte Packing5/2
  Bus Creator2/1 -> Bus Creator/2  "Cell02"
  Bus Creator5/1 -> Bus Creator/7  "Cell07"
  Byte Packing8/1 -> Bus Creator9/4  "Cell11_charge"
  Byte Packing1/1 -> Bus Creator2/4  "Cell2_charge"
  Bus Creator10/1 -> Bus Creator/12  "Cell12"
  Bus Creator8/1 -> Bus Creator/10  "Cell10"
  EtherCAT PDO Receive28/1 -> Byte Packing6/1
  Byte Packing3/1 -> Bus Creator4/4  "Cell6_charge"
  EtherCAT PDO Receive13/1 -> Byte Packing3/1
  EtherCAT PDO Receive16/1 -> Bus Creator4/2  "Cell6_voltage"
  EtherCAT PDO Receive51/1 -> Bus Creator14/1  "Cell4_status"
  EtherCAT PDO Receive05/1 -> Bus Creator2/2  "Cell2_voltage"
  EtherCAT PDO Receive06/1 -> Bus Creator2/3  "Cell2_current"
  EtherCAT PDO Receive25/1 -> Bus Creator6/1  "Cell8_status"
  EtherCAT PDO Receive31/1 -> Bus Creator7/2  "Cell9_voltage"
  Byte Packing12/1 -> Bus Creator13/4  "Cell3_charge"
  Byte Packing/1 -> Bus Creator1/4  "Cell1_charge"
  EtherCAT PDO Receive38/1 -> Byte Packing8/1
  EtherCAT PDO Receive50/1 -> Byte Packing13/2
  Bus Creator3/1 -> Bus Creator/5  "Cell05"
  EtherCAT PDO Receive22/1 -> Bus Creator5/3  "Cell7_current"
  Byte Packing9/1 -> Bus Creator10/4  "Cell12_charge"
  Byte Packing5/1 -> Bus Creator6/4  "Cell8_charge"
  Bus Creator1/1 -> Bus Creator/1  "Cell01"
  EtherCAT PDO Receive36/1 -> Bus Creator8/2  "Cell10_voltage"
  EtherCAT PDO Receive07/1 -> Byte Packing1/1
  EtherCAT PDO Receive47/1 -> Bus Creator10/3  "Cell12_current"
  EtherCAT PDO Receive10/1 -> Byte Packing2/1
  EtherCAT PDO Receive20/1 -> Bus Creator5/1  "Cell7_status"
  EtherCAT PDO Receive42/1 -> Bus Creator9/3  "Cell11_current"
  EtherCAT PDO Receive02/1 -> Bus Creator1/3  "Cell1_current"
  EtherCAT PDO Receive34/1 -> Byte Packing7/2
  EtherCAT PDO Receive2/1 -> Bus Creator2/1  "Cell2_status"
  Bus Creator/1 -> Data/1
  EtherCAT PDO Receive03/1 -> Byte Packing/1
  EtherCAT PDO Receive08/1 -> Byte Packing1/2
